simulink model "state_observability"  (R2014a)
settings: Solver=ode45  StartTime=0.0  StopTime=t_sim  RelTol=absTol  AbsTol=relTol
undefined symbols (not defined in the file): omega_B, omega_bias_I, q_init, r_ref_I
libraries: lib_gyro_fusion x3
settings Model: Creator=kirill  LastModifiedBy=kirill

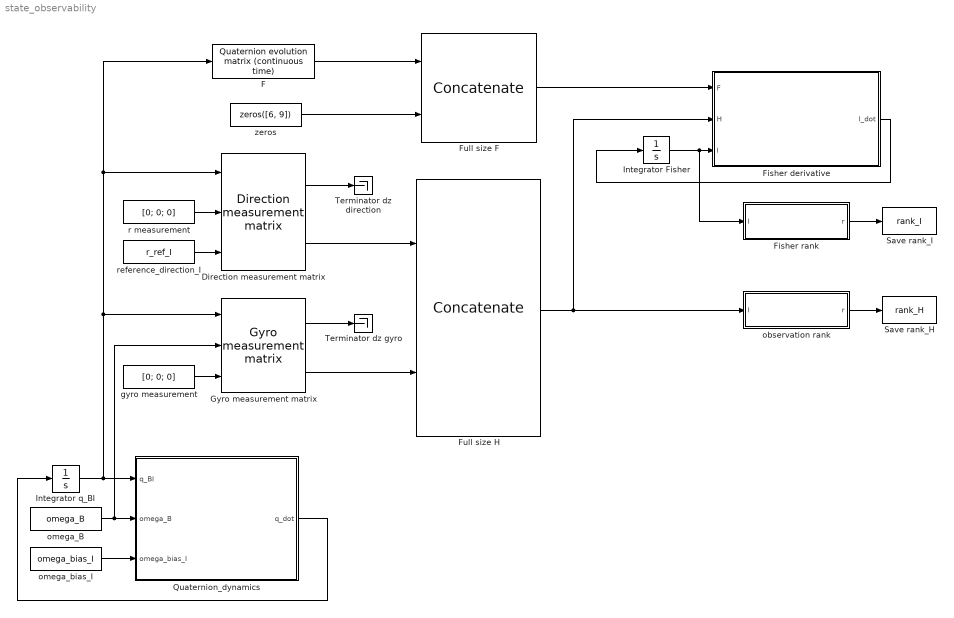
== system state_observability ==
  Direction measurement matrix : lib_gyro_fusion/Direction measurement matrix
  F : lib_gyro_fusion/Kalman predictor/Quaternion evolution matrix (continuous time)
  Fisher derivative : MATLAB Function  TreatAsAtomicUnit=on
  Fisher rank : MATLAB Function  TreatAsAtomicUnit=on
  Full size F : Concatenate  Mode=Multidimensional array
  Full size H : Concatenate  Mode=Multidimensional array
  Gyro measurement matrix : lib_gyro_fusion/Gyro measurement matrix
  Integrator Fisher : Integrator  InitialCondition=zeros(9)
  Integrator q_BI : Integrator  InitialCondition=q_init
  Quaternion_dynamics : MATLAB Function  TreatAsAtomicUnit=on
  Save rank_H : ToWorkspace  VariableName=rank_H  SaveFormat=Timeseries  SampleTime=-1
  Save rank_I : ToWorkspace  VariableName=rank_I  SaveFormat=Timeseries  SampleTime=-1
  Terminator dz direction : Terminator
  Terminator dz gyro : Terminator
  gyro measurement : Constant  Value=[0; 0; 0]
  observation rank : MATLAB Function  TreatAsAtomicUnit=on
  omega_B : Constant  Value=omega_B
  omega_bias_I : Constant  Value=omega_bias_I
  r measurement : Constant  Value=[0; 0; 0]
  reference_direction_I : Constant  Value=r_ref_I
  zeros : Constant  Value=zeros([6, 9])
  wires:
  omega_B/1 -> Gyro measurement matrix/2, Quaternion_dynamics/2(omega_B)
  omega_bias_I/1 -> Quaternion_dynamics/3(omega_bias_I)
  Quaternion_dynamics/1(q_dot) -> Integrator q_BI/1
  Integrator q_BI/1 -> Quaternion_dynamics/1(q_BI), Gyro measurement matrix/1, Direction measurement matrix/1, F/1
  F/1 -> Full size F/1
  zeros/1 -> Full size F/2
  Full size F/1 -> Fisher derivative/1(F)
  Integrator Fisher/1 -> Fisher rank/1(I), Fisher derivative/3(I)
  Fisher derivative/1(I_dot) -> Integrator Fisher/1
  Full size H/1 -> observation rank/1(I), Fisher derivative/2(H)
  Direction measurement matrix/1 -> Terminator dz direction/1
  Gyro measurement matrix/1 -> Terminator dz gyro/1
  Direction measurement matrix/2 -> Full size H/1
  Gyro measurement matrix/2 -> Full size H/2
  reference_direction_I/1 -> Direction measurement matrix/3
  Fisher rank/1(r) -> Save rank_I/1
  gyro measurement/1 -> Gyro measurement matrix/3
  r measurement/1 -> Direction measurement matrix/2
  observation rank/1(r) -> Save rank_H/1

== matlab function state_observability/Fisher derivative ==
  data: I_dot output; F input; H input; I input
function I_dot = fisher_dynamics(F, H, I)
%#codegen

I_dot = -F' * I - I * F + H' * H;

== matlab function state_observability/observation rank ==
  data: I input; r output
function r = rank_fisher(I)
%#codegen
r = rank(I);

== matlab function state_observability/Fisher rank ==
  data: I input; r output
function r = rank_fisher(I)
%#codegen
r = rank(I);

== matlab function state_observability/Quaternion_dynamics ==
  data: q_dot output; q_BI input; omega_B input; omega_bias_I input
function q_dot = qiuat_dynamics(q_BI, omega_B, omega_bias_I)
%#codegen
q_dot = poissonRHS(0, q_BI, omega_B, omega_bias_I);
